simulink model "test_dcmotor"  (R2021a)
settings: Solver=VariableStepAuto  StartTime=0.0  StopTime=10.0  FixedStep=0.01  RelTol=1e-3
libraries: fl_lib x9, ee_lib x6, nesl_utility x5
settings Model: Creator=beave  LastModifiedBy=thana
settings SolverCC: AlgebraicLoopSolver=TrustRegion
settings DebuggingCC: SFMachineParentedDataDiag=warning

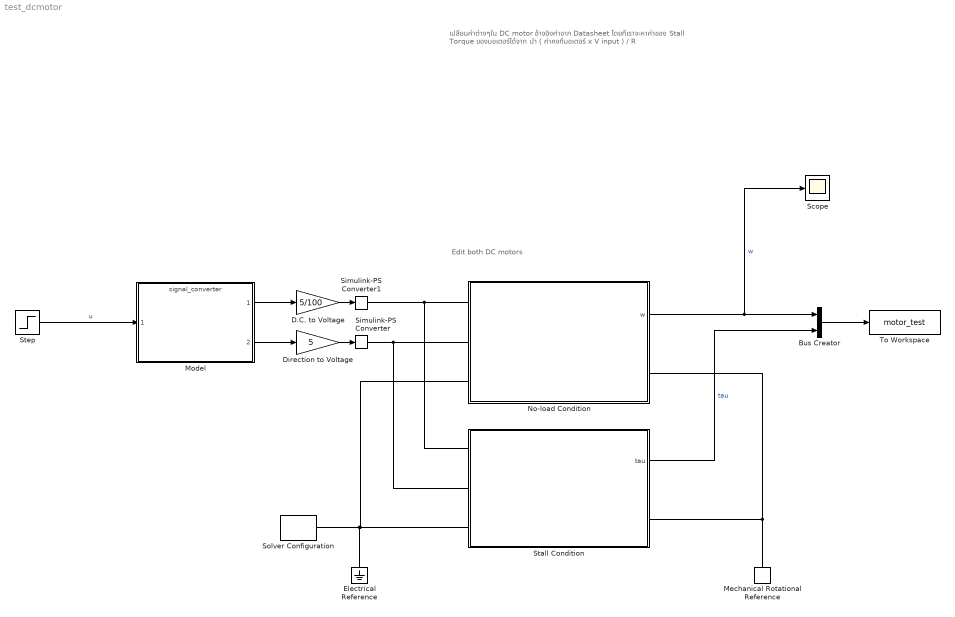
== system test_dcmotor ==
  note: เปลี่ยนค่าต่างๆใน DC motor อ้างอิงค่าจาก Datasheet
      | โดยที่เราจะหาค่าของ Stall Torque ของมอเตอร์ได้จาก
      | นำ ( ค่าคงที่มอเตอร์ x V input ) / R
  note: Edit both DC motors
  Bus Creator : BusCreator  Inputs=2
  D.C. to Voltage : Gain  Gain=5/100
  Direction to Voltage : Gain  Gain=5
  Electrical Reference : fl_lib/Electrical/Electrical Elements/Electrical Reference
  Mechanical Rotational Reference : fl_lib/Mechanical/Rotational Elements/Mechanical Rotational Reference
  Model : ModelReference  ModelNameDialog=signal_converter.slx  SimulationMode=Normal  ModelReferenceVersion=2.1
  No-load Condition : Subsystem
  Scope : Scope
  Simulink-PS Converter : nesl_utility/Simulink-PS Converter  PhysicalDomain=network_engine_domain  SubClassName=ps_input  LeftPortType=input  RightPortType=output  PseudoPeriodic=off  Frequencies=[]  NoiseDistribution=none  NoiseParameters=[]  Unit=1  AffineConversion=off  FilteringAndDerivatives=provide  SimscapeFilterOrder=1  InputFilterTimeConstant=0.001  UdotUserProvided=0
      settings: SourceProductBaseCode=PW,SS
  Simulink-PS Converter1 : nesl_utility/Simulink-PS Converter  PhysicalDomain=network_engine_domain  SubClassName=ps_input  LeftPortType=input  RightPortType=output  PseudoPeriodic=off  Frequencies=[]  NoiseDistribution=none  NoiseParameters=[]  Unit=1  AffineConversion=off  FilteringAndDerivatives=provide  SimscapeFilterOrder=1  InputFilterTimeConstant=0.001  UdotUserProvided=0
      settings: SourceProductBaseCode=PW,SS
  Solver Configuration : nesl_utility/Solver Configuration  PhysicalDomain=network_engine_domain  SubClassName=solver  LeftPortType=input  RightPortType=generic  Tones=[]  Harmonics=[]  SimulateNoise=off  Profile=off  UseLocalSampling=off  EnableSwitchedLinearOptims=on  FrequencyDomain=off  UseCCode=off  RelTol=0.001  AbsTol=1e-06  MinStep=1e-09  ToWorkspace=off  RevertToSquareIcSolve=off  NumHomotopyIterations=100  PhasorMode=off  PhasorModeNumHarmonics=1  DoDC=off  ResidualTolerance=1e-09  UseLocalSolver=off  LocalSolverChoice=NE_BACKWARD_EULER_ADVANCER  LocalSolverSampleTime=0.001  DoFixedCost=off  MaxNonlinIter=3  MaxModeIter=2  ComputeImpulses=off  ImpulseIterations=2  LinearAlgebra=auto  EquationFormulation=NE_TIME_EF  DelaysMemoryBudget=1024  AutomaticFiltering=on  FilteringTimeConstant=0.001  PartitionStorageMethod=AS_NEEDED  PartitionMemoryBudget=1024  PartitionMethod=ROBUST
      settings: SourceProductBaseCode=PW,SS
  Stall Condition : Subsystem
  Step : Step  After=120  SampleTime=0
  To Workspace : ToWorkspace  VariableName=motor_test  SaveFormat=Timeseries  SampleTime=-1
  wires:
  D.C. to Voltage/1 -> Simulink-PS Converter1/1
  Direction to Voltage/1 -> Simulink-PS Converter/1
  Step/1 -> Model/1  "u"
  Model/1 -> D.C. to Voltage/1
  Model/2 -> Direction to Voltage/1
  No-load Condition/1(w) -> Scope/1, Bus Creator/1  "w"
  Stall Condition/1(tau) -> Bus Creator/2  "tau"
  Bus Creator/1 -> To Workspace/1
  connections:
  Solver Configuration/RConn1 -- No-load Condition/LConn3 -- Stall Condition/LConn3 -- Electrical Reference/LConn1
  Simulink-PS Converter1/RConn1 -- No-load Condition/LConn1 -- Stall Condition/LConn1
  Simulink-PS Converter/RConn1 -- No-load Condition/LConn2 -- Stall Condition/LConn2
  Mechanical Rotational Reference/LConn1 -- No-load Condition/RConn1 -- Stall Condition/RConn1

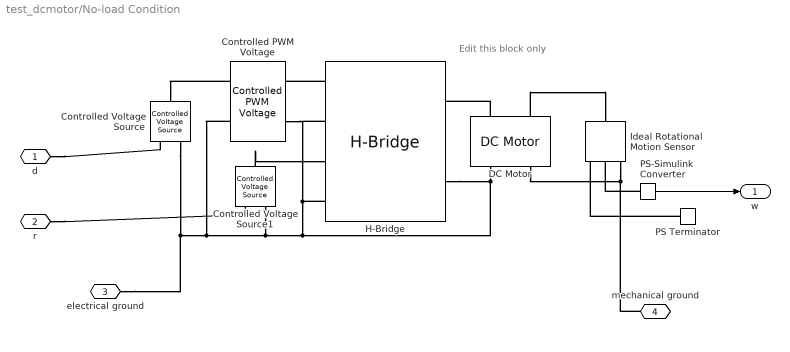
== system test_dcmotor/No-load Condition ==
  note: Edit this block only
  Controlled PWM Voltage : ee_lib/Integrated Circuits/Controlled PWM Voltage  F=1000 Hz  TD=0 s  pulse_width_offset=0 s  pulse_min=0 s  Vmin=0 V  Vmax=5 V  Vm=5 V  pwm_or_av=2  event_type=1  sample_time=1e-6 s  u_min=0  u_max=1
  Controlled Voltage Source : fl_lib/Electrical/Electrical Sources/Controlled Voltage Source
  Controlled Voltage Source1 : fl_lib/Electrical/Electrical Sources/Controlled Voltage Source
  DC Motor : ee_lib/Electromechanical/Brushed Motors/DC Motor  field_option=ee.enum.field_option.pm  Rf=100 Ohm  Lf=1 H  Laf=0.15 H  If0=0 A  parameterization=ee.enum.dcparam_option.torque_speed  Ra=3.9 Ohm  La=0.01 H  emf_or_torque=ee.enum.emf_or_torque.kv  Kv=0.072e-3 V/rpm  Ki=6.876e-4 N*m/A  T_stall="0.7032509651565111  N*m"  w_max=6850 rpm  w_rated=15000 rpm  P_rated=0.08 W  V_rated=12 V  J=0.1 g*cm^2  lam_param=ee.enum.lam_param.current  lam=0 N*m/(rad/s)  i_noload=2 A  V_i_noload=1.5 V  speed0=0 rpm  enable_fault_armature=ee.enum.faults.faultEnable.no  rev_faulted=1 / 3  G_faulted_armature=1e-5 S  fault_trigger_armature=ee.enum.faults.faultTrigger.temporal  t_fault_armature=1 s  max_permissible_current_armature=inf A  t_fail_on_current_armature=1 s  enable_fault_field=ee.enum.faults.faultEnable.no  G_faulted_field=1e-5 S  fault_trigger_field=ee.enum.faults.faultTrigger.temporal  t_fault_field=1 s  max_permissible_current_field=inf A  t_fail_on_current_field=1 s  fault_action=ee.enum.faults.faultAction.none  alpha=3.93e-3 1/K  Tmeas=25 degC  thermal_mass=100 J/K  initial_temperature=25 degC
  H-Bridge : ee_lib/Semiconductors & Converters/Converters/H-Bridge  supply_ports=ee.enum.supply_ports.hidesupply  Venable=2.5 V  Vmax=12 V  Vreverse=2.5 V  Vbrake=2.5 V  Vm=12 V  pwm_or_av=ee.enum.pwm_or_av.pwm  regenerative_braking_mode=ee.enum.converters.regenerative_braking_mode.depends_on_rev  discontinuous=ee.enum.current_profile.continuous  freewheeling_mode=ee.enum.converters.freewheeling_mode.one_switch_one_diode  Ron=1e-8 Ohm  Don=1e-8 Ohm  Goff=1e-8 S  Rload=10 Ohm  Lload=1e-5 H  F=10 kHz  thermal_mass=100 J/K  initial_temperature=298.15 K  Ron2=0.1 Ohm  Don2=0.05 Ohm  Tmeas=298.15 K  Tmeas2=398.15 K
  Ideal Rotational Motion Sensor : fl_lib/Mechanical/Mechanical Sensors/Ideal Rotational Motion Sensor  wrap_angle=simscape.enum.onoff.off  offset=0 rad
  PS Terminator : fl_lib/Physical Signals/Sinks/PS Terminator
  PS-Simulink Converter : nesl_utility/PS-Simulink Converter  PhysicalDomain=network_engine_domain  SubClassName=ps_output  LeftPortType=input  RightPortType=output  PseudoPeriodic=off  Frequencies=[]  Unit=inherit  AffineConversion=off
      settings: SourceProductBaseCode=PW,SS
  d : PMIOPort  Side=Left
  r : PMIOPort  Port=2  Side=Left
  electrical ground : PMIOPort  Port=3  Side=Left
  mechanical ground : PMIOPort  Port=4  Side=Right
  w : Outport
  wires:
  PS-Simulink Converter/1 -> w/1
  connections:
  PS Terminator/LConn1 -- Ideal Rotational Motion Sensor/RConn3
  DC Motor/LConn1 -- H-Bridge/RConn1
  Controlled Voltage Source/RConn2 -- electrical ground/RConn1 -- Controlled PWM Voltage/LConn2 -- Controlled Voltage Source1/RConn2 -- Controlled PWM Voltage/RConn2 -- H-Bridge/LConn2 -- H-Bridge/LConn4 -- DC Motor/RConn1 -- H-Bridge/RConn2
  Controlled PWM Voltage/LConn1 -- Controlled Voltage Source/LConn1
  Ideal Rotational Motion Sensor/RConn1 -- DC Motor/RConn2 -- mechanical ground/RConn1
  DC Motor/LConn2 -- Ideal Rotational Motion Sensor/LConn1
  PS-Simulink Converter/LConn1 -- Ideal Rotational Motion Sensor/RConn2
  H-Bridge/LConn1 -- Controlled PWM Voltage/RConn1
  Controlled Voltage Source1/LConn1 -- H-Bridge/LConn3
  d/RConn1 -- Controlled Voltage Source/RConn1
  r/RConn1 -- Controlled Voltage Source1/RConn1

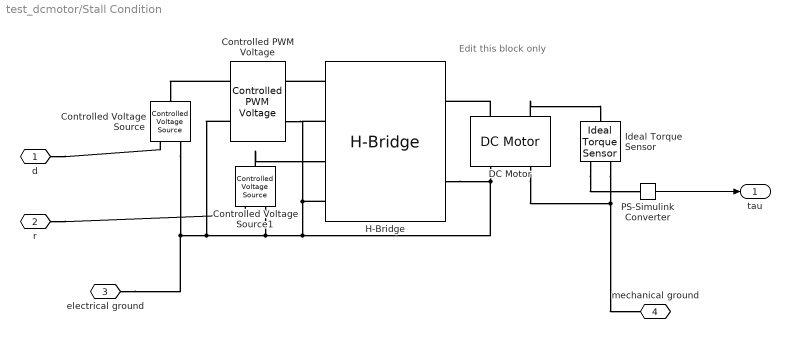
== system test_dcmotor/Stall Condition ==
  note: Edit this block only
  Controlled PWM Voltage : ee_lib/Integrated Circuits/Controlled PWM Voltage  F=1000 Hz  TD=0 s  pulse_width_offset=0 s  pulse_min=0 s  Vmin=0 V  Vmax=5 V  Vm=5 V  pwm_or_av=2  event_type=1  sample_time=1e-6 s  u_min=0  u_max=1
  Controlled Voltage Source : fl_lib/Electrical/Electrical Sources/Controlled Voltage Source
  Controlled Voltage Source1 : fl_lib/Electrical/Electrical Sources/Controlled Voltage Source
  DC Motor : ee_lib/Electromechanical/Brushed Motors/DC Motor  field_option=ee.enum.field_option.pm  Rf=100 Ohm  Lf=1 H  Laf=0.15 H  If0=0 A  parameterization=ee.enum.dcparam_option.torque_speed  Ra=3.9 Ohm  La=0.01 H  emf_or_torque=ee.enum.emf_or_torque.kv  Kv=0.072e-3 V/rpm  Ki=6.876e-4 N*m/A  T_stall="0.7032509651565111  N*m"  w_max=6850 rpm  w_rated=15000 rpm  P_rated=0.08 W  V_rated=12 V  J=0.1 g*cm^2  lam_param=ee.enum.lam_param.current  lam=0 N*m/(rad/s)  i_noload=2 A  V_i_noload=1.5 V  speed0=0 rpm  enable_fault_armature=ee.enum.faults.faultEnable.no  rev_faulted=1 / 3  G_faulted_armature=1e-5 S  fault_trigger_armature=ee.enum.faults.faultTrigger.temporal  t_fault_armature=1 s  max_permissible_current_armature=inf A  t_fail_on_current_armature=1 s  enable_fault_field=ee.enum.faults.faultEnable.no  G_faulted_field=1e-5 S  fault_trigger_field=ee.enum.faults.faultTrigger.temporal  t_fault_field=1 s  max_permissible_current_field=inf A  t_fail_on_current_field=1 s  fault_action=ee.enum.faults.faultAction.none  alpha=3.93e-3 1/K  Tmeas=25 degC  thermal_mass=100 J/K  initial_temperature=25 degC
  H-Bridge : ee_lib/Semiconductors & Converters/Converters/H-Bridge  supply_ports=ee.enum.supply_ports.hidesupply  Venable=2.5 V  Vmax=12 V  Vreverse=2.5 V  Vbrake=2.5 V  Vm=12 V  pwm_or_av=ee.enum.pwm_or_av.pwm  regenerative_braking_mode=ee.enum.converters.regenerative_braking_mode.depends_on_rev  discontinuous=ee.enum.current_profile.continuous  freewheeling_mode=ee.enum.converters.freewheeling_mode.one_switch_one_diode  Ron=1e-8 Ohm  Don=1e-8 Ohm  Goff=1e-8 S  Rload=10 Ohm  Lload=1e-5 H  F=10 kHz  thermal_mass=100 J/K  initial_temperature=298.15 K  Ron2=0.1 Ohm  Don2=0.05 Ohm  Tmeas=298.15 K  Tmeas2=398.15 K
  Ideal Torque Sensor : fl_lib/Mechanical/Mechanical Sensors/Ideal Torque Sensor
  PS-Simulink Converter : nesl_utility/PS-Simulink Converter  PhysicalDomain=network_engine_domain  SubClassName=ps_output  LeftPortType=input  RightPortType=output  PseudoPeriodic=off  Frequencies=[]  Unit=inherit  AffineConversion=off
      settings: SourceProductBaseCode=PW,SS
  d : PMIOPort  Side=Left
  r : PMIOPort  Port=2  Side=Left
  electrical ground : PMIOPort  Port=3  Side=Left
  mechanical ground : PMIOPort  Port=4  Side=Right
  tau : Outport
  wires:
  PS-Simulink Converter/1 -> tau/1
  connections:
  r/RConn1 -- Controlled Voltage Source1/RConn1
  Controlled Voltage Source1/LConn1 -- H-Bridge/LConn3
  H-Bridge/LConn1 -- Controlled PWM Voltage/RConn1
  Ideal Torque Sensor/RConn1 -- DC Motor/RConn2 -- mechanical ground/RConn1
  electrical ground/RConn1 -- Controlled Voltage Source/RConn2 -- Controlled PWM Voltage/LConn2 -- Controlled Voltage Source1/RConn2 -- H-Bridge/LConn4 -- H-Bridge/LConn2 -- Controlled PWM Voltage/RConn2 -- DC Motor/RConn1 -- H-Bridge/RConn2
  DC Motor/LConn1 -- H-Bridge/RConn1
  Ideal Torque Sensor/RConn2 -- PS-Simulink Converter/LConn1
  d/RConn1 -- Controlled Voltage Source/RConn1
  DC Motor/LConn2 -- Ideal Torque Sensor/LConn1
  Controlled PWM Voltage/LConn1 -- Controlled Voltage Source/LConn1
